simulink model "RightArmAgent"  (Simulink 6.5)
settings: Solver=ode45  SolverMode=SingleTasking  StartTime=0.0  StopTime=10.0  RelTol=1e-3  AbsTol=1e-6
settings Model: Creator=The MathWorks Inc.  LastModifiedBy=suarezjl  ExtModeTrigMode=oneshot  ExtModeArmWhenConnect=off  ExtModeAutoUpdateStatusClock=off
settings DataIOCC: LimitDataPoints=off  SignalLoggingName=logsOut
settings OptimizationCC: BooleanDataType=off  InlineInvariantSignals=on
settings DebuggingCC: CheckExecutionContextPreStartOutputMsg=on  CheckExecutionContextRuntimeOutputMsg=on  SolverPrmCheckMsg=none  MultiTaskDSMMsg=warning  MultiTaskCondExecSysMsg=none  IntegerOverflowMsg=none  StrictBusMsg=None
settings HardwareCC: TargetUnknown=on
settings ModelReferenceCC: UpdateModelReferenceTargets=IfOutOfDate
settings RTWCC: IncludeERTFirstTime=on

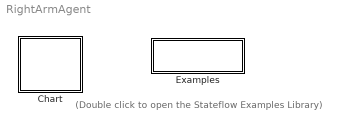
== system RightArmAgent ==
  note: (Double click to open the
      | Stateflow Examples Library)
  Chart : Stateflow chart
  Examples : Subsystem
      settings: OpenFcn=sf('Private','sf_examples')
      mask Display: disp('Examples')

== system RightArmAgent/Examples ==

== stateflow chart Chart ==
  state InitialArmRoutine
    Hungerforce\CogDemo\RightArm\HomingController.ComputeHomingPressures()
    Hungerforce\CogDemo\RightArm\SampleIndPressure.HW_IO_6()
    Hungerforce\CogDemo\RightArm\StateMachine.Wait(50)
  state InitializeFunctions
    Hungerforce\CogDemo\RightArm\HomingController.Initial()
    Hungerforce\CogDemo\RightArm\SampleIndPressure.Initialize()
    Hungerforce\CogDemo\RightArm\PIDNonLinCtrl.Initial()
    Hungerforce\CogDemo\RightArm\ForwardKinematics.Initialize()
    Hungerforce\CogDemo\RightArm\InverseKinematics.Initialize()
    Hungerforce\CogDemo\RightArm\SampleIndPressure.Disable_ZMasking()
  state WriteHomeDesiredLogicalAngles
    Hungerforce\CogDemo\RightArm\SampleIndPressure.Enable_ZMasking()
    Hungerforce\CogDemo\RightArm\SampleIndPressure.WriteHomePositions()
  state LoadHomePosition
    Hungerforce\CogDemo\RightArm\SampleIndPressure.HW_IO_6()
    Hungerforce\CogDemo\RightArm\PIDNonLinCtrl.PID_NonLin_6Press()
    Hungerforce\CogDemo\RightArm\ForwardKinematics.ForwardKinematics()
    Hungerforce\CogDemo\RightArm\InverseKinematics.InverseKinematics()
  state PID_NonLinCtrlLoop
    Hungerforce\CogDemo\RightArm\Filter.FilterDesiredAngles()
    Hungerforce\CogDemo\RightArm\PIDNonLinCtrl.PID_NonLin_12Press()
    Hungerforce\CogDemo\RightArm\SampleIndPressure.HW_IO_12()
    Hungerforce\CogDemo\RightArm\PIDNonLinCtrl.Read_CurrentPressure()
    Hungerforce\CogDemo\RightArm\ForwardKinematics.ForwardKinematics()
    Hungerforce\CogDemo\RightArm\InverseKinematics.InverseKinematics()
    Hungerforce\CogDemo\RightArm\StateMachine.Wait(50)
  (default) -> InitializeFunctions : Start
  InitialArmRoutine -> InitialArmRoutine [order 1] : Default
  InitializeFunctions -> InitialArmRoutine : Always
  WriteHomeDesiredLogicalAngles -> LoadHomePosition : Always
  LoadHomePosition -> PID_NonLinCtrlLoop : Always
  InitialArmRoutine -> WriteHomeDesiredLogicalAngles [order 2] : Signal="Go to next state"
  PID_NonLinCtrlLoop -> PID_NonLinCtrlLoop : Default
